simulink model "PSOAV"  (R2019a)
settings: Solver=VariableStepAuto  StartTime=0.0  StopTime=10.0  RelTol=1e-6
libraries: powerlib x11, re_lib x2, powerlib_meascontrol x1
settings Model: Creator=user
settings DataIOCC: ReturnWorkspaceOutputs=off
settings DebuggingCC: ArithmeticOperatorsInVariantConditions=warning

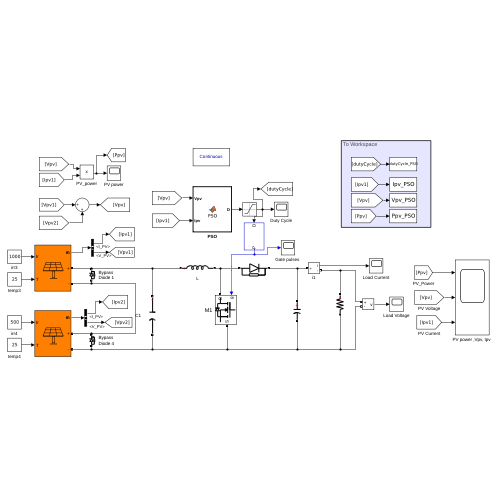
[thumbnail: Simulink's stored preview of the top-level diagram]
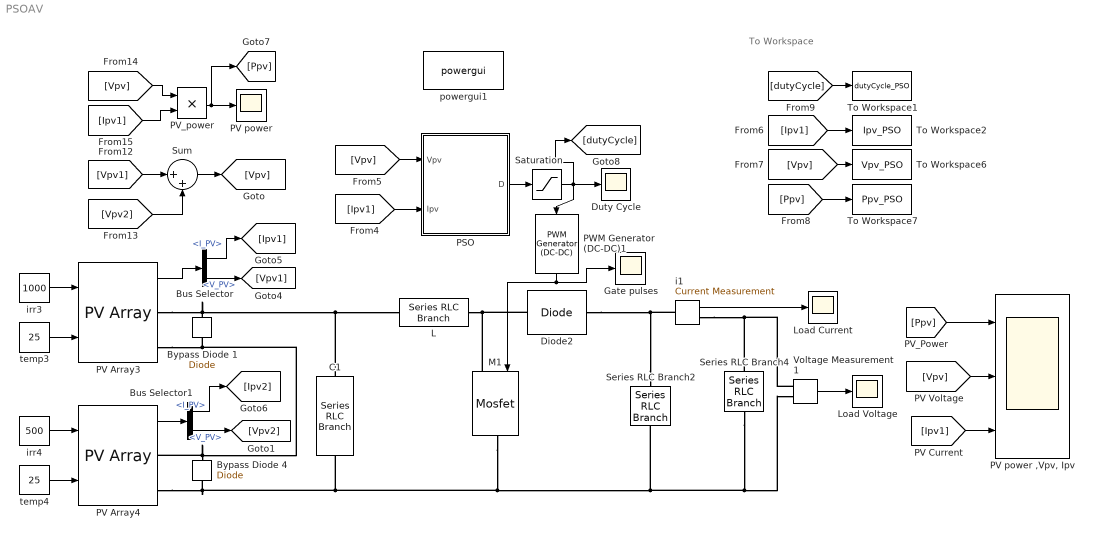
== system PSOAV ==
  note: To Workspace
  Bus Selector : BusSelector  OutputSignals=I_PV,V_PV
  Bus Selector1 : BusSelector  OutputSignals=I_PV,V_PV
  Bypass Diode 1 : powerlib/Power Electronics/Diode  Ron=0.001  Lon=0  Vf=0.8  IC=0  UseSnubber=off  Rs=500  Cs=250e-9  Measurements=off
  Bypass Diode 4 : powerlib/Power Electronics/Diode  Ron=0.001  Lon=0  Vf=0.8  IC=0  UseSnubber=off  Rs=500  Cs=250e-9  Measurements=off
  C1 : powerlib/Elements/Series RLC Branch  LConnTagsString=__new0  RConnTagsString=__new0  BranchType=C  Resistance=0.0001  Inductance=1e-3  SetiL0=off  InitialCurrent=0  Capacitance=1e-3  Setx0=on  InitialVoltage=0  Measurements=None
  Diode2 : powerlib/Power Electronics/Diode  Ron=0.001  Lon=0  Vf=0.8  IC=0  UseSnubber=0  Rs=500  Cs=250e-9  Measurements=off
  Duty Cycle : Scope
  "Gate pulses " : Scope
  L : powerlib/Elements/Series RLC Branch  LConnTagsString=__new0  RConnTagsString=__new0  BranchType=L  Resistance=1e-3  Inductance=1.1478e-3  SetiL0=off  InitialCurrent=0  Capacitance=1e-6  Setx0=off  InitialVoltage=0  Measurements=None
  Load Current : Scope
  Load Voltage : Scope
  M1 : powerlib/Power Electronics/Mosfet  Ron=1e-3  Lon=0  Rd=1e-3  Vfd=0  IC=0  Rs=inf  Cs=inf  Measurements=off
  PSO : MATLAB Function  TreatAsAtomicUnit=on
  PV Array3 : re_lib/Solar/PV Array  Npar=1  Nser=1  PlotType=one module @ 25 deg.C & specified irradiances  S_vec="[ 1000  500  100 ]"  Temp_C_vec="[ 45 25  ]"  ModuleName=User-defined  PlotWhenSelected=off  Pm=213.15  Ncell=60  Voc=36.3  Isc=7.84  Vm=29  Im=7.35  beta_Voc_pc=-0.36099  alpha_Isc_pc=0.102  beta_Voc=-0.13104  alpha_Isc=0.0079968  IL=7.8654  I0=2.9273e-10  nI=0.98119  Rsh=313.0553  Rs=0.39381  RobustModel=off  RobustCellTemperature=313.3991  BAL=off  Tc=1e-6  Tfilter=5e-5
  PV Array4 : re_lib/Solar/PV Array  Npar=1  Nser=1  PlotType=array @ 1000 W/m2 & specified temperatures  S_vec="[ 1000  500  100 ]"  Temp_C_vec="[ 45 25  ]"  ModuleName=User-defined  PlotWhenSelected=off  Pm=213.15  Ncell=60  Voc=36.3  Isc=7.84  Vm=29  Im=7.35  beta_Voc_pc=-0.36099  alpha_Isc_pc=0.102  beta_Voc=-0.13104  alpha_Isc=0.0079968  IL=7.8654  I0=2.9273e-10  nI=0.98119  Rsh=313.0553  Rs=0.39381  RobustModel=off  RobustCellTemperature=313.3991  BAL=off  Tc=1e-6  Tfilter=5e-5
  PV power : Scope
  "PV power ,Vpv, Ipv " : Scope  NumInputPorts=3
  PV_power : Product
  PWM Generator (DC-DC)1 : powerlib_meascontrol/Pulse & Signal Generators/PWM Generator (DC-DC)  Fsw=5e3  Ts=0
  Saturation : Saturate  UpperLimit=0.75  LowerLimit=0.3
  Series RLC Branch2 : powerlib/Elements/Series RLC Branch  LConnTagsString=__new0  RConnTagsString=__new0  BranchType=C  Resistance=1e-4  Inductance=200e-6  SetiL0=off  InitialCurrent=0  Capacitance=3227e-6  Setx0=off  InitialVoltage=40  Measurements=None
  Series RLC Branch4 : powerlib/Elements/Series RLC Branch  LConnTagsString=__new0  RConnTagsString=__new0  BranchType=R  Resistance=100  Inductance=200e-6  SetiL0=off  InitialCurrent=0  Capacitance=1000e-6  Setx0=off  InitialVoltage=40  Measurements=None
  Sum : Sum  Inputs=|++
  To Workspace1 : ToWorkspace  VariableName=dutyCycle_PSO  SampleTime=-1
  To Workspace2 : ToWorkspace  VariableName=Ipv_PSO  SampleTime=-1
  To Workspace6 : ToWorkspace  VariableName=Vpv_PSO  SampleTime=-1
  To Workspace7 : ToWorkspace  VariableName=Ppv_PSO  SampleTime=-1
  Voltage Measurement1 : powerlib/Measurements/Voltage Measurement  PhasorSimulation=off  OutputType=Magnitude  PSBequivalent=0
  i1 : powerlib/Measurements/Current Measurement  PhasorSimulation=off  OutputType=Magnitude  PSBequivalent=0
  irr3 : Constant  Value=1000
  irr4 : Constant  Value=500
  powergui1 : powerlib/powergui  Priority=1  SimulationMode=Continuous  SampleTime=50e-6  frequency=60  Iterations=50  frequencyindice=0  Pbase=100e6  ErrMax=1e-4  UnitsV=kV  UnitsW=MW  buscounter=0  FunctionMessages=off  echomessages=off  EnableUseOfTLC=off  CurrentSourceSwitches=off  DisableSnubberDevices=off  DisableRonSwitches=off  DisableVfSwitches=off  DisplayEquations=off  AutomaticDiscreteSolvers=off  SolverType=Tustin/Backward Euler (TBE)  Interpol=off  ExternalGateDelay=off  methode=off  Ts=100  x0status=blocks  SPID=on  SwTol=0  HookPort=off  NonlinearTolerance=1e-4  nMaxIteration=100  ContinueOnMaxIteration=off  RestoreLinks=warning  ResistiveCurrentMeasurement=off  Frange=[0:2:500]  Ylog=off  Xlog=on  ShowGrid=off  save=off  variable=ZData  structure=0  ZoomFFT=off  StartTime=0.0  cycles=1  DisplayStyle=1  fundamental=60  FreqAxis=off  MaxFrequency=1000  frequencyindicesteady=1  RmsSteady=1  display=off
  temp3 : Constant  Value=25
  temp4 : Constant  Value=25
  wires:
  [Ipv1] -> PSO/2(Ipv)
  temp3/1 -> PV Array3/2
  [Vpv] -> To Workspace6/1
  irr4/1 -> PV Array4/1
  [Vpv2] -> Sum/2
  temp4/1 -> PV Array4/2
  Bus Selector/2 -> [Vpv1]  "<V_PV>"
  [Vpv1] -> Sum/1
  Bus Selector/1 -> [Ipv1]  "<I_PV>"
  [Ipv1] -> PV_power/2
  Bus Selector1/1 -> [Ipv2]  "<I_PV>"
  Voltage Measurement1/1 -> Load Voltage/1
  [dutyCycle] -> To Workspace1/1
  PV Array3/1 -> Bus Selector/1
  PWM Generator (DC-DC)1/1 -> "Gate pulses "/1, M1/1
  [Ppv] -> To Workspace7/1
  [Vpv] -> PV_power/1
  [Vpv] -> PSO/1(Vpv)
  Bus Selector1/2 -> [Vpv2]  "<V_PV>"
  irr3/1 -> PV Array3/1
  PV Array4/1 -> Bus Selector1/1
  Sum/1 -> [Vpv]
  [Ipv1] -> To Workspace2/1
  PSO/1(D) -> Saturation/1
  Saturation/1 -> PWM Generator (DC-DC)1/1, [dutyCycle], Duty Cycle/1
  PV_power/1 -> PV power/1, [Ppv]
  i1/1 -> Load Current/1
  [Ipv1] -> "PV power ,Vpv, Ipv "/3
  [Vpv] -> "PV power ,Vpv, Ipv "/2
  [Ppv] -> "PV power ,Vpv, Ipv "/1
  connections:
  C1/LConn1 -- L/LConn1 -- Bypass Diode 1/RConn1 -- PV Array3/RConn1
  Bypass Diode 4/RConn1 -- PV Array4/RConn1 -- PV Array3/RConn2 -- Bypass Diode 1/LConn1
  Bypass Diode 4/LConn1 -- PV Array4/RConn2 -- Voltage Measurement1/LConn2 -- Series RLC Branch4/RConn1 -- Series RLC Branch2/RConn1 -- M1/RConn1 -- C1/RConn1
  Series RLC Branch4/LConn1 -- Voltage Measurement1/LConn1 -- i1/RConn1
  M1/LConn1 -- L/RConn1 -- Diode2/LConn1
  Series RLC Branch2/LConn1 -- i1/LConn1 -- Diode2/RConn1

== matlab function PSOAV/PSO ==
  settings: updateMethod=DISCRETE  sampleTime=1e-4
  data: Vpv input; D output; Ipv input
function D = PSO(Vpv,Ipv)

persistent u;
persistent dcurrent;
persistent pbest;
persistent p;            %power
persistent dc;           %duty cycle
persistent v;            %velocity
persistent counter;
persistent gbest;
% initialization :
if(isempty(counter))
    counter=0;          
    dcurrent=0.5;       %current duty cycle
    gbest=0.5;
    p=zeros(3,1);       %power
    v=zeros(3,1);       %voltage
    pbest=zeros(3,1);
    u=0;                
    dc=zeros(3,1);      %duty cycle
    %initial dc for each particle
    dc(1)=0.2;
    dc(2)=0.4;
    dc(3)=0.7;
    
end

% AT the first time , this if ignored (counter=0)
%Delay
if(counter>=1 && counter<300)
    D=dcurrent;
    counter=counter+1;
    return;                 %return control to the invoking function before it reaches the end of the function.
end
counter=0;                  %reset the counter 

%calculate the fittnes function (power) of each particle,
%then compare the current value of the function with previous one 
%if the current value is better than the previous ,update the value 
%Note: at the first time , this if ignored (u=0)
if(u>=1 && u<=3)
    if((Vpv*Ipv)>p(u))
        p(u)=Vpv*Ipv;
        pbest(u)=dcurrent;
    end
end


u=u+1;
% AT the first time , this if excuted  because it consist the condition...
% u==0(initial value of u)
if(u==5)
    u=1;
end

if(u==1)
    D=dc(u);
    dcurrent=D;
    counter=1;
    return;
elseif(u==2)
    D=dc(u);
    dcurrent=D;
    counter=1;
    return;
elseif(u==3)
    D=dc(u);
    dcurrent=D;
    counter=1;
    return;
elseif(u==4 )
    [m,i]=max(p);       %finds the indices of the maximum values of P (max power)and returns them in output vector i
    gbest=pbest(i);     % find the location(duty) of the particle which has max P 
    D=gbest;
    dcurrent=D;
    counter=1;
    %update velocity and duty cycle
    v(1)=updatevelocity(v(1),pbest(1),dc(1),gbest)
    v(2)=updatevelocity(v(2),pbest(2),dc(2),gbest)
    v(3)=updatevelocity(v(3),pbest(3),dc(3),gbest)
    
    %update duty cycle
    dc(1)=updateduty(dc(1),v(1))
    dc(2)=updateduty(dc(2),v(2))
    dc(3)=updateduty(dc(3),v(3))
    
    
    return;
    
else %if u==0 
   
    D=0.1;
    
end


end
function vfinal=updatevelocity(velocity,pobest,d,gwbest)
% PSO Parameters
w=0.4;
c1=1.2;         % Personal Learning Coefficient
c2=2;           % Global Learning Coefficient

vfinal = (w*velocity)+(c1*rand(1)*(pobest-d))+(c2*rand(1)*(gwbest-d));
end
function dfinal=updateduty(d,velocity)
dup=d+velocity;
if(dup>1)
    dfinal=1;
elseif(dup<0)
    dfinal=0;
else
    dfinal=dup;
end
end
